simulink model "flatsat_data_send_2018"  (R2018b)
settings: Solver=VariableStepAuto  StartTime=0.0  StopTime=Inf  RelTol=1e-3
values from neighbouring files (symbols this model uses):
  t_send = 1/25    (= 0.04)    [flatsat_data_send_init.m]
undefined symbols (not defined in the file or in its folder): serial
libraries: instrumentlib x2
settings Model: EnablePacing=on  Creator=Alex Zhen  LastModifiedBy=Alex Zhen

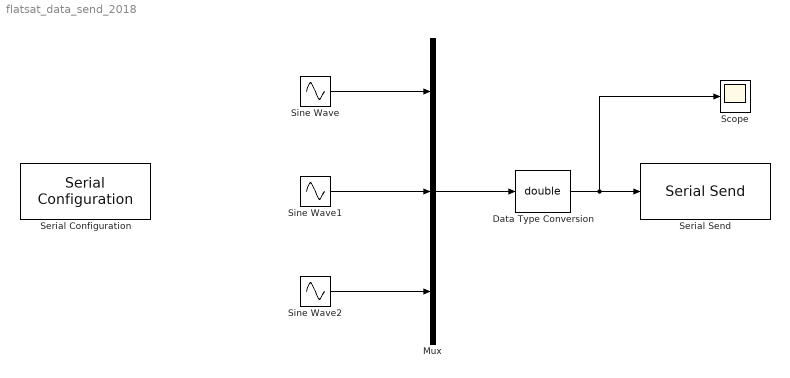
== system flatsat_data_send_2018 ==
  Data Type Conversion : DataTypeConversion  OutDataTypeStr=double  LockScale=on
  Mux : Mux  Inputs=3
  Scope : Scope
  Serial Configuration : instrumentlib/Serial Configuration  Priority=-200000  ComPortMenu=COM9  ComPort=COM9  ObjConstructor=serial('COM9');  BaudRate=115200  DataBits=8  Parity=none  StopBits=1  FlowControl=none  Timeout=10  ByteOrder=LittleEndian
  Serial Send : instrumentlib/Serial Send  ComPortMenu=COM9  ComPort=COM9  ObjConstructor=serial('COM9');  Terminator=<none>  EnableBlockingMode=on
  Sine Wave : Sin  SampleTime=t_send
  Sine Wave1 : Sin  Amplitude=2  Frequency=2  SampleTime=t_send
  Sine Wave2 : Sin  Amplitude=3  Frequency=3  SampleTime=t_send
  wires:
  Sine Wave1/1 -> Mux/2
  Sine Wave2/1 -> Mux/3
  Sine Wave/1 -> Mux/1
  Mux/1 -> Data Type Conversion/1
  Data Type Conversion/1 -> Scope/1, Serial Send/1
